simulink model "actuator_study"  (R2021b)
settings: Solver=VariableStepAuto  StartTime=0.0  StopTime=10  RelTol=1e-3
values from neighbouring files (symbols this model uses):
  G_1 = [ mot_eff,mot_eff,mot_eff,mot_eff;0,-12.8,0,12.8;2.7,0,-2.7,0;-0.115,0.115,-0.115,0.115]./conv    [Model_Parameters.m]    (also in wls_test.m)
  G_2 = [0,0,0,0;0,0,0,0;0,0,0,0;-0.06,0.06,-0.06,0.06]./conv    [Model_Parameters.m]    (also in wls_test.m)
  H_z_den = [1]    [Model_Parameters.m]
  H_z_num = [1]    [Model_Parameters.m]
  Hz2rads = 6.28    [Model_Parameters.m]    (also in wls_test.m)
  M = 0.1*1/(1-exp(-20*Ts))    [Model_Parameters.m]
  mot_den = [1]    [Model_Parameters.m]
  mot_num = [1]    [Model_Parameters.m]
  pseudo_g12 = pinv(G_1+G_2)    [Model_Parameters.m]    (also in wls_test.m)
  Ts = 1/500    (= 0.002)    [Model_Parameters.m]
libraries: dspsrcs4 x3, simulink x1
settings Model: Creator=tomasodeponti  LastModifiedBy=tomasodeponti

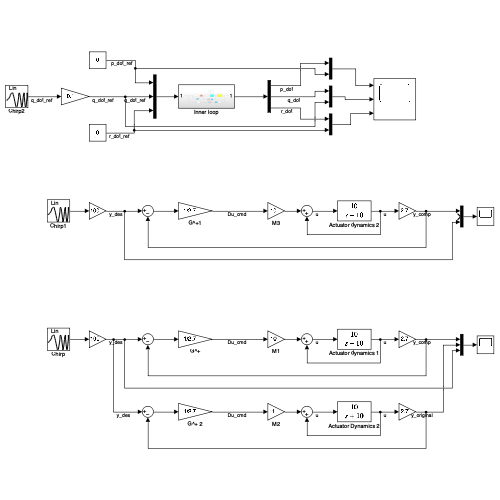
[thumbnail: Simulink's stored preview of the top-level diagram]
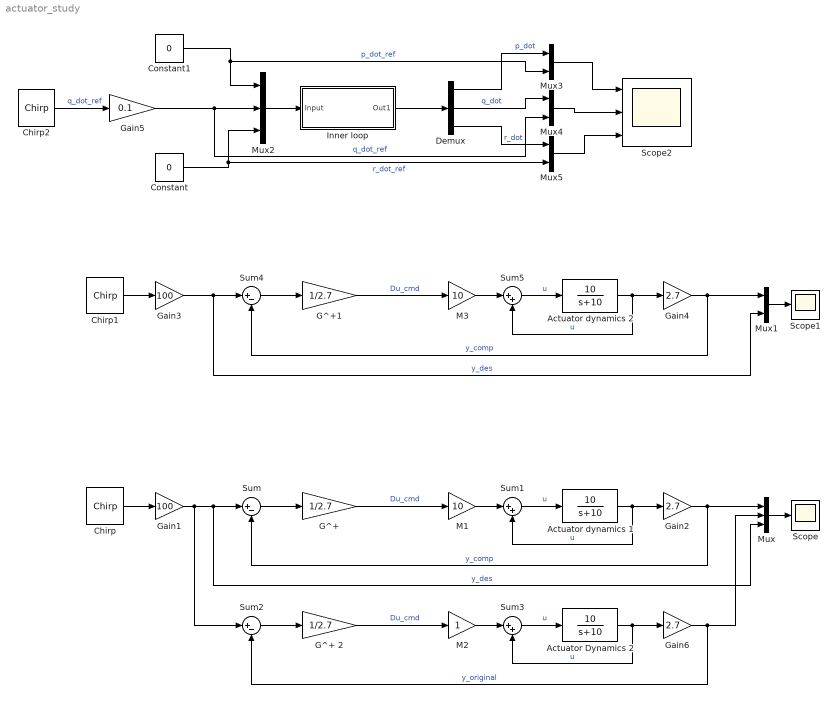
== system actuator_study ==
  Actuator Dynamics 2 : TransferFcn  Numerator=[10]  Denominator=[1 10]
  Actuator dynamics 1 : TransferFcn  Numerator=[10]  Denominator=[1 10]
  Actuator dynamics 2 : TransferFcn  Numerator=[10]  Denominator=[1 10]
  Chirp : dspsrcs4/Chirp  sweep=Linear  mode=Unidirectional  f0=0.1  f1=0.5  t1=1  Tsweep=10  phase=0  Ts=1/8000  spf=1  datatype=Double  OutputFrames=off
  Chirp1 : dspsrcs4/Chirp  sweep=Linear  mode=Unidirectional  f0=0.1  f1=0.5  t1=1  Tsweep=10  phase=0  Ts=1/8000  spf=1  datatype=Double  OutputFrames=off
  Chirp2 : dspsrcs4/Chirp  sweep=Linear  mode=Unidirectional  f0=0.1  f1=0.5  t1=1  Tsweep=10  phase=0  Ts=Ts  spf=1  datatype=Double  OutputFrames=off
  Constant : Constant  Value=0
  Constant1 : Constant  Value=0
  Demux : Demux  Outputs=3
  G^+ : Gain  Gain=1/2.7
  G^+ 2 : Gain  Gain=1/2.7
  G^+1 : Gain  Gain=1/2.7
  Gain1 : Gain  Gain=100
  Gain2 : Gain  Gain=2.7
  Gain3 : Gain  Gain=100
  Gain4 : Gain  Gain=2.7
  Gain5 : Gain  Gain=0.1
  Gain6 : Gain  Gain=2.7
  Inner loop : Subsystem
  M1 : Gain  Gain=10
  M2 : Gain
  M3 : Gain  Gain=10
  Mux : Mux  Inputs=3
  Mux1 : Mux  Inputs=3
  Mux2 : Mux  Inputs=3
  Mux3 : Mux  Inputs=2
  Mux4 : Mux  Inputs=2
  Mux5 : Mux  Inputs=2
  Scope : Scope
  Scope1 : Scope
  Scope2 : Scope  NumInputPorts=3
  Sum : Sum  Inputs=|+-
  Sum1 : Sum  Inputs=|++
  Sum2 : Sum  Inputs=|+-
  Sum3 : Sum  Inputs=|++
  Sum4 : Sum  Inputs=|+-
  Sum5 : Sum  Inputs=|++
  wires:
  Chirp/1 -> Gain1/1
  Gain1/1 -> Sum2/1, Sum/1, Mux/3  "y_des"
  Sum/1 -> G^+/1
  G^+/1 -> M1/1  "Du_cmd"
  Sum1/1 -> Actuator dynamics 1/1  "u"
  Gain2/1 -> Mux/1, Sum/2  "y_comp"
  Mux/1 -> Scope/1
  Actuator dynamics 1/1 -> Sum1/2, Gain2/1  "u"
  M1/1 -> Sum1/1
  Sum3/1 -> Actuator Dynamics 2/1  "u"
  M2/1 -> Sum3/1
  Actuator Dynamics 2/1 -> Sum3/2, Gain6/1  "u"
  G^+ 2/1 -> M2/1  "Du_cmd"
  Sum2/1 -> G^+ 2/1
  Gain6/1 -> Mux/2, Sum2/2  "y_original"
  M3/1 -> Sum5/1
  Actuator dynamics 2/1 -> Sum5/2, Gain4/1  "u"
  Chirp1/1 -> Gain3/1
  G^+1/1 -> M3/1  "Du_cmd"
  Sum4/1 -> G^+1/1
  Sum5/1 -> Actuator dynamics 2/1  "u"
  Mux1/1 -> Scope1/1
  Gain4/1 -> Mux1/1, Sum4/2  "y_comp"
  Gain3/1 -> Sum4/1, Mux1/3  "y_des"
  Constant1/1 -> Mux2/1, Mux3/2  "p_dot_ref"
  Constant/1 -> Mux2/3, Mux5/2  "r_dot_ref"
  Mux2/1 -> Inner loop/1(Input)
  Gain5/1 -> Mux4/2, Mux2/2  "q_dot_ref"
  Inner loop/1(Out1) -> Demux/1
  Demux/1 -> Mux3/1  "p_dot"
  Demux/2 -> Mux4/1  "q_dot"
  Demux/3 -> Mux5/1  "r_dot"
  Mux3/1 -> Scope2/1
  Mux4/1 -> Scope2/2
  Mux5/1 -> Scope2/3
  Chirp2/1 -> Gain5/1  "q_dot_ref"

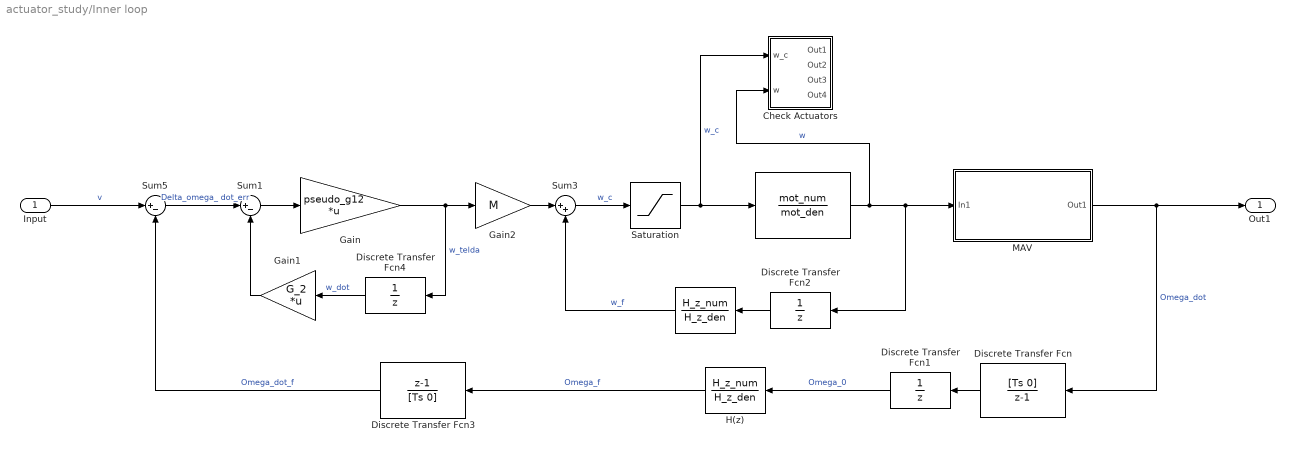
== system actuator_study/Inner loop ==
  Input : Inport  PortDimensions=3
  " " : DiscreteTransferFcn  Numerator=H_z_num  Denominator=H_z_den  DenCoefDataTypeStr=int16
      mask Display: disp('H(z)')
  "  " : DiscreteTransferFcn  Numerator=mot_num  Denominator=mot_den  DenCoefDataTypeStr=int16
      mask Display: disp('A(z)')
  Check Actuators : Subsystem
  Discrete Transfer Fcn : DiscreteTransferFcn  Numerator=[Ts 0]  Denominator=[1 -1]
  Discrete Transfer Fcn1 : DiscreteTransferFcn  Denominator=[1 0]
  Discrete Transfer Fcn2 : DiscreteTransferFcn  Denominator=[1 0]
  Discrete Transfer Fcn3 : DiscreteTransferFcn  Numerator=[1 -1]  Denominator=[Ts 0]
  Discrete Transfer Fcn4 : DiscreteTransferFcn  Denominator=[1 0]
  Gain : Gain  Gain=pseudo_g12  Multiplication=Matrix(K*u)
      mask Display: disp('(G1+G2)^+','texmode','on')
  Gain1 : Gain  Gain=G_2  Multiplication=Matrix(K*u)
      mask Display: disp('G2')
  Gain2 : Gain  Gain=M
      mask Display: disp('M')
  H(z) : DiscreteTransferFcn  Numerator=H_z_num  Denominator=H_z_den  DenCoefDataTypeStr=int16
      mask Display: disp('H(z)')
  MAV : Subsystem
      mask Display:
      | %image('C:\Users\Tomaso\Pictures\Screenshots\Screenshot 2021-12-02 165056.png'); % Use "Edit Image" on toolstrip to change.
      | disp('MAV')
  Saturation : Saturate  UpperLimit=150*Hz2rads  LowerLimit=0
  Sum1 : Sum  Inputs=|+-
  Sum3 : Sum  Inputs=|++
  Sum5 : Sum  Inputs=|+-
  Out1 : Outport  PortDimensions=3
  wires:
  "  "/1 -> Check Actuators/2(w), Discrete Transfer Fcn2/1, MAV/1(In1)  "w"
  Discrete Transfer Fcn/1 -> Discrete Transfer Fcn1/1
  Discrete Transfer Fcn1/1 -> H(z)/1  "Omega_0"
  Discrete Transfer Fcn2/1 -> " "/1
  Saturation/1 -> Check Actuators/1(w_c), "  "/1  "w_c"
  " "/1 -> Sum3/2  "w_f"
  H(z)/1 -> Discrete Transfer Fcn3/1  "Omega_f"
  Discrete Transfer Fcn3/1 -> Sum5/2  "Omega_dot_f"
  Gain/1 -> Discrete Transfer Fcn4/1, Gain2/1  "w_telda"
  Sum5/1 -> Sum1/1  "Delta_omega_ dot_err"
  Sum1/1 -> Gain/1
  Discrete Transfer Fcn4/1 -> Gain1/1  "w_dot"
  Gain1/1 -> Sum1/2
  Input/1 -> Sum5/1  "v"
  Gain2/1 -> Sum3/1
  Sum3/1 -> Saturation/1  "w_c"
  MAV/1(Out1) -> Discrete Transfer Fcn/1, Out1/1  "Omega_dot"

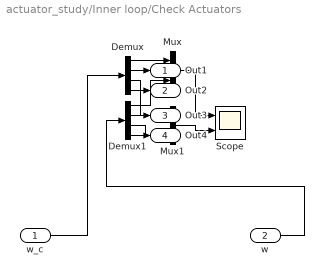
== system actuator_study/Inner loop/Check Actuators ==
  w_c : Inport
  w : Inport  Port=2
  Demux : Demux
  Demux1 : Demux
  Mux : Mux  Inputs=2
  Mux1 : Mux  Inputs=2
  Scope : Scope  NumInputPorts=2
  Out1 : Outport
  Out2 : Outport  Port=2
  Out3 : Outport  Port=3
  Out4 : Outport  Port=4
  wires:
  Demux1/3 -> Mux1/2
  w_c/1 -> Demux/1
  Demux1/4 -> Out4/1
  Demux/2 -> Out1/1
  w/1 -> Demux1/1
  Demux/4 -> Out2/1
  Mux/1 -> Scope/1
  Demux/3 -> Mux1/1
  Demux1/1 -> Mux/2
  Demux/1 -> Mux/1
  Mux1/1 -> Scope/2
  Demux1/2 -> Out3/1

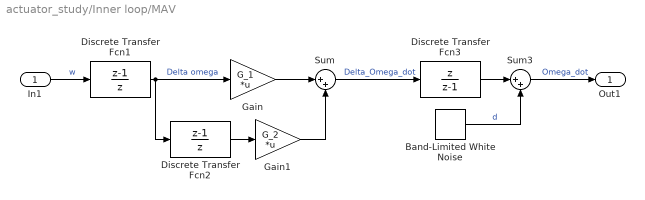
== system actuator_study/Inner loop/MAV ==
  In1 : Inport  PortDimensions=4
  Band-Limited White Noise : simulink/Sources/Band-Limited White Noise  Cov=[0.00000001]  Ts=Ts  seed=[23341]
  Discrete Transfer Fcn1 : DiscreteTransferFcn  Numerator=[1 -1]  Denominator=[1 0]
  Discrete Transfer Fcn2 : DiscreteTransferFcn  Numerator=[1 -1]  Denominator=[1 0]
  Discrete Transfer Fcn3 : DiscreteTransferFcn  Numerator=[1 0]  Denominator=[1 -1]
  Gain : Gain  Gain=G_1  Multiplication=Matrix(K*u)
      mask Display: disp('G1')
  Gain1 : Gain  Gain=G_2  Multiplication=Matrix(K*u)
      mask Display: disp('G2')
  Sum : Sum  Inputs=|++
  Sum3 : Sum  Inputs=|++
  Out1 : Outport  PortDimensions=3
  wires:
  In1/1 -> Discrete Transfer Fcn1/1  "w"
  Discrete Transfer Fcn1/1 -> Discrete Transfer Fcn2/1, Gain/1  "Delta omega"
  Discrete Transfer Fcn2/1 -> Gain1/1
  Gain/1 -> Sum/1
  Gain1/1 -> Sum/2
  Sum/1 -> Discrete Transfer Fcn3/1  "Delta_Omega_dot"
  Discrete Transfer Fcn3/1 -> Sum3/1
  Band-Limited White Noise/1 -> Sum3/2  "d"
  Sum3/1 -> Out1/1  "Omega_dot"
